simulink model "ue_tracking"  (R2020a)
settings: Solver=FixedStepDiscrete  StartTime=0.0  StopTime=300  FixedStep=system.step  RelTol=1e-3
undefined symbols (not defined in the file or in its folder): frame, physconst, system, UE
libraries: commsync2 x3, phasedtxrxlib x3, phaseddoalib x2, commsink2 x2, commdigbbndpm3 x2, commfilt2 x2, commsequence2 x2, phasedbflib x2, commchan3 x2, dspsrcs4 x1, commrfcorlib x1, commutil2 x1
settings Model: PauseTimes=500  NumberOfSteps=10  Creator=jose_  LastModifiedBy=jose_
settings DebuggingCC: ReadBeforeWriteMsg=DisableAll  WriteAfterWriteMsg=DisableAll  WriteAfterReadMsg=DisableAll  MultiTaskDSMMsg=none
settings ModelReferenceCC: UpdateModelReferenceTargets=IfOutOfDate
settings SFSimCC: SFSimEcho=off

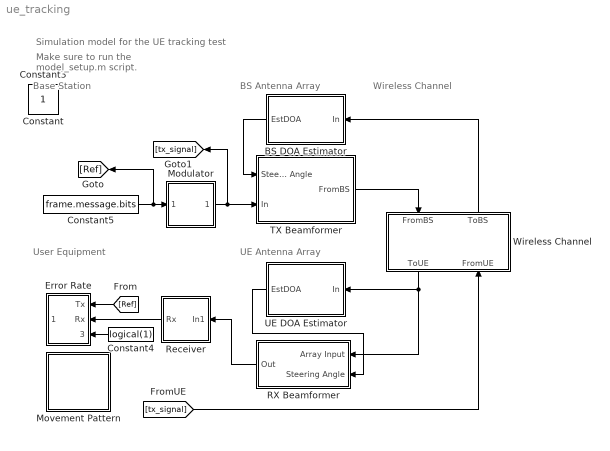
== system ue_tracking ==
  note: UE Antenna Array
  note: BS Antenna Array
  note: Wireless Channel
  note: User Equipment
  note: Base Station
  note: Make sure to run the model_setup.m script.
  note: Simulation model for the UE tracking test
  BS DOA Estimator : Subsystem
      mask Display: image('$imagefile'); % Use "Edit Image" on toolstrip to change.
  Constant4 : Constant  Value=logical(1)
  Constant5 : Constant  Value=frame.message.bits  SampleTime=system.step
  Error Rate : Subsystem
  Modulator : Subsystem
      mask Display: image('$imagefile'); % Use "Edit Image" on toolstrip to change.
  Movement Pattern : Subsystem
      mask Display: image('$imagefile'); % Use "Edit Image" on toolstrip to change.
  RX Beamformer : Subsystem
      mask Display: image('$imagefile'); % Use "Edit Image" on toolstrip to change.
  Receiver : Subsystem
      mask Display: image('$imagefile'); % Use "Edit Image" on toolstrip to change.
  TX Beamformer : Subsystem
      mask Display: image('$imagefile'); % Use "Edit Image" on toolstrip to change.
  UE DOA Estimator : Subsystem
      mask Display: image('$imagefile'); % Use "Edit Image" on toolstrip to change.
  Wireless Channel : Subsystem
      settings: PortSchema="{\"entries\":[{\"content\":{\"sides\":[{\"content\":{\"connectorIds\":[]},\"type\":\"ConnectorPlacement.EquallySpacedRectSide\",\"uuid\":\"75bf1423-5319-4e93-9a5f-3cb48862b48c\"},{\"content\":{\"connectorIds\":[],\"side\":\"RIGHT\"},\"type\":\"ConnectorPlacement.EquallySpacedRectSide\",\"uuid\":\"e5a97bb0-755e-4af0-92a4-b9cdae2be643\"},{\"content\":{\"connectorIds\":[\"In1\",\"Out2\"],\"side\":\"TOP\"},\"type\":\"ConnectorPlacement.EquallySpacedRectSide\",\"uuid\":\"177e5c48-1e85-4698-92ad-7f86d2203077\"},{\"content\":{\"connectorIds\":[\"Out1\",\"In2\"],\"side\":\"BOTTOM\"},\"type\":\"ConnectorPlacement.EquallySpacedRectSide\",\"uuid\":\"6d25e01a-df39-4651-afd4-30d22a581838\"}]},\"type\":\"ConnectorPlacement.EquallySpacedConnector\",\"uuid\":\"14e51280-45ab-4234-928d-dd2548344928\"}],\"packageUris\":[\"http://schema.mathworks.com/mf0/Connector/19700101\"],\"version\":\"1.0\"}"
      mask Display: image('$imagefile'); % Use "Edit Image" on toolstrip to change.
  Constant : Constant  IOType=siggen
  Constant3 : Constant  IOType=siggen
  wires:
  RX Beamformer/1(Out) -> Receiver/1(In1)
  Wireless Channel/2(ToBS) -> BS DOA Estimator/1(In)
  [tx_signal] -> Wireless Channel/2(FromUE)
  BS DOA Estimator/1(EstDOA) -> TX Beamformer/1(Steering Angle)
  Constant4/1 -> Error Rate/3(Rst)
  [Ref] -> Error Rate/1(Tx)
  Constant5/1 -> Modulator/1(Message), [Ref]
  Modulator/1(Out1) -> [tx_signal], TX Beamformer/2(In)
  Wireless Channel/1(ToUE) -> UE DOA Estimator/1(In), RX Beamformer/1(Array Input)
  Receiver/1(Rx) -> Error Rate/2(Rx)
  TX Beamformer/1(FromBS) -> Wireless Channel/1(FromBS)
  UE DOA Estimator/1(EstDOA) -> RX Beamformer/2(Steering Angle)

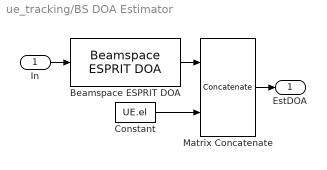
== system ue_tracking/BS DOA Estimator ==
  In : Inport
  Beamspace ESPRIT DOA : phaseddoalib/Beamspace ESPRIT DOA  PropagationSpeed=physconst( 'LightSpeed' )  OperatingFrequency=system.freq  NumSignalsSource=Property  NumSignalsMethod=AIC  NumSignals=1  SpatialSmoothing=0  Method=TLS  BeamFanCenter=0  NumBeamsSource=Auto  NumBeams=2  SimulateUsing=Code generation  SensorArray=AntennaArray
      settings: SourceProductBaseCode=AR
  Constant : Constant  Value=UE.el
  Matrix Concatenate : Concatenate  Mode=Multidimensional array
  EstDOA : Outport
  wires:
  In/1 -> Beamspace ESPRIT DOA/1
  Beamspace ESPRIT DOA/1 -> Matrix Concatenate/1
  Matrix Concatenate/1 -> EstDOA/1
  Constant/1 -> Matrix Concatenate/2

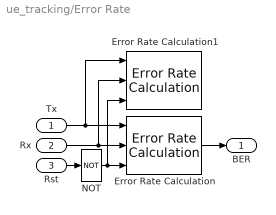
== system ue_tracking/Error Rate ==
  Tx : Inport
  Rx : Inport  Port=2
  Rst : Inport  Port=3
  Error Rate Calculation : commsink2/Error Rate Calculation  N=0  st_delay=0  cp_mode=Entire frame  subframe=[]  PMode=Port  WsName=ErrorVec  RsMode2=on  stop=off  numErr=100  maxBits=1e6
  Error Rate Calculation1 : commsink2/Error Rate Calculation  N=0  st_delay=0  cp_mode=Entire frame  subframe=[]  PMode=Workspace  WsName=ErrorVec  RsMode2=on  stop=off  numErr=100  maxBits=1e6
  NOT : Logic  Operator=NOT  IconShape=distinctive  AllPortsSameDT=off  OutDataTypeStr=boolean
  BER : Outport
  wires:
  Tx/1 -> Error Rate Calculation1/1, Error Rate Calculation/1
  Rx/1 -> Error Rate Calculation1/2, Error Rate Calculation/2
  Error Rate Calculation/1 -> BER/1
  Rst/1 -> NOT/1
  NOT/1 -> Error Rate Calculation1/3, Error Rate Calculation/3

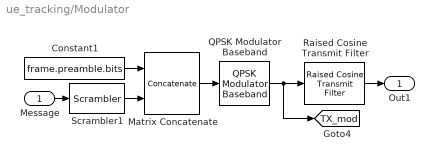
== system ue_tracking/Modulator ==
  Message : Inport
  Constant1 : Constant  Value=frame.preamble.bits  SampleTime=system.step
  Matrix Concatenate : Concatenate  Mode=Multidimensional array
  QPSK Modulator Baseband : commdigbbndpm3/QPSK Modulator Baseband  InType=Bit  Enc=Gray  Ph=system.mod.PhaseOffset  outDtype=double  outWordLen=16  outUDDataType=sfix(16)  outFracLenMode=Best precision  outFracLen=15  outDataTypeStr=double  outLastDataTypeStr=double
  Raised Cosine Transmit Filter : commfilt2/Raised Cosine Transmit Filter  filtType=Square root  R=system.tx.rc.rolloff  filtSpan=system.tx.rc.span  N=system.tx.rc.interpolation  filterGain=sqrt(system.tx.rc.interpolation)  InputProcessing=Columns as channels (frame based)  RateOptions=Enforce single-rate processing  framing=Mute  checkCoeff=off  variableName=rcTxFilt  checkGain=Normalized  sampMode=Mute  saveAsFlag=0  currentFiltSpan=system.tx.rc.span  D=(system.tx.rc.span)/2  launchFVT=on  roundingMode=Floor  overflowMode=off  coeffDataTypeStr=Inherit: Same word length as input  coeffMin=[]  coeffMax=[]  coeffLastDataTypeStr=Inherit: Same word length as input  outputDataTypeStr=Inherit: Same as accumulator  outputMin=[]  outputMax=[]  outputLastDataTypeStr=Inherit: Same as accumulator
  Scrambler1 : commsequence2/Scrambler  M=2  poly=[1 1 1 0 1]  iniStaSource=Dialog Parameter  ini_sta=[0 0 0 0]  resetViaPort=off
      settings: SourceProductBaseCode=CM
  Out1 : Outport
  tag scope: TX_mod=global
  wires:
  QPSK Modulator Baseband/1 -> [TX_mod], Raised Cosine Transmit Filter/1
  Matrix Concatenate/1 -> QPSK Modulator Baseband/1
  Raised Cosine Transmit Filter/1 -> Out1/1
  Constant1/1 -> Matrix Concatenate/1
  Message/1 -> Scrambler1/1
  Scrambler1/1 -> Matrix Concatenate/2

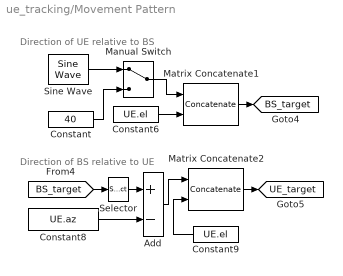
== system ue_tracking/Movement Pattern ==
  note: Direction of BS relative to UE
  note: Direction of UE relative to BS
  Add : Sum  Inputs=+-
  Constant : Constant  Value=40
  Constant6 : Constant  Value=UE.el  VectorParams1D=off
  Constant8 : Constant  Value=UE.az
  Constant9 : Constant  Value=UE.el  VectorParams1D=off
  Manual Switch : ManualSwitch
  Matrix Concatenate1 : Concatenate  Mode=Multidimensional array
  Matrix Concatenate2 : Concatenate  Mode=Multidimensional array
  Selector : Selector  InputPortWidth=2  IndexOptions=Index vector (dialog)  Indices=1  OutputSizes=1
  Sine Wave : dspsrcs4/Sine Wave  Amplitude=UE.max_ang  Frequency=UE.movement_freq  Phase=0  SampleMode=Discrete  OutComplex=Real  CompMethod=Table lookup  TableSize=Speed  SampleTime=system.step  SamplesPerFrame=1  ResetState=Restart at time zero  OutputFrames=off  dataType=double  wordLen=16  udDataType=sfix(16)  fracBitsMode=Best precision  numFracBits=15  OutDataTypeStr=double  LastOutDataTypeStr=double
  tag scope: BS_target=global, UE_target=global
  wires:
  Constant6/1 -> Matrix Concatenate1/2
  [BS_target] -> Selector/1
  Constant8/1 -> Add/2
  Matrix Concatenate2/1 -> [UE_target]
  Constant9/1 -> Matrix Concatenate2/2
  Matrix Concatenate1/1 -> [BS_target]
  Sine Wave/1 -> Manual Switch/1
  Constant/1 -> Manual Switch/2
  Manual Switch/1 -> Matrix Concatenate1/1
  Selector/1 -> Add/1
  Add/1 -> Matrix Concatenate2/1

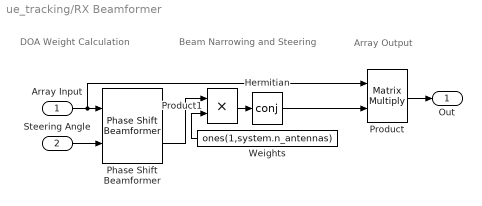
== system ue_tracking/RX Beamformer ==
  note: Beam Narrowing and Steering
  note: DOA Weight Calculation
  note: Array Output
  Array Input : Inport
  Steering Angle : Inport  Port=2
  Hermitian : Math  Operator=conj  SaturateOnIntegerOverflow=on
  Phase Shift Beamformer : phasedbflib/Phase Shift Beamformer  PropagationSpeed=physconst( 'LightSpeed' )  OperatingFrequency=system.freq  DirectionSource=Input port  Direction=[ 0; 0 ]  NumPhaseShifterBits=0  WeightsNormalization=Preserve power  WeightsOutputPort=on  SimulateUsing=Code generation  SensorArray=AntennaArray
      settings: SourceProductBaseCode=AR
  Product : Product  Multiplication=Matrix(*)
  Product1 : Product
  Weights : Constant  Value=ones(1,system.n_antennas)
  Out : Outport
  wires:
  Product1/1 -> Hermitian/1
  Hermitian/1 -> Product/2
  Product/1 -> Out/1
  Weights/1 -> Product1/2
  Phase Shift Beamformer/2 -> Product1/1
  Array Input/1 -> Product/1, Phase Shift Beamformer/1
  Steering Angle/1 -> Phase Shift Beamformer/2

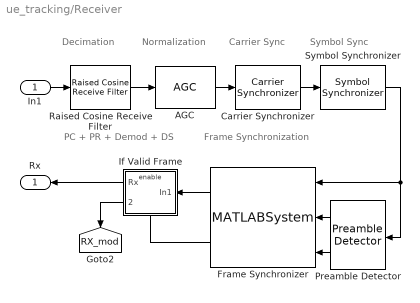
== system ue_tracking/Receiver ==
  note: PC + PR + Demod + DS
  note: Frame Synchronization
  note: Symbol Sync
  note: Carrier Sync
  note: Normalization
  note: Decimation
  In1 : Inport
  AGC : commrfcorlib/AGC  LegacyMode=off  DetectorMethod=Rectifier  LoopMethod=Linear  UpdatePeriod=100  StepSize=0.1  AdaptationStepSize=system.rx.agc.step  DesiredOutputPower=system.rx.agc.output_power  AveragingLength=system.rx.agc.average_length  MaximumGain=30  MaxPowerGain=system.rx.agc.max_power  GainOutputPort=off  InputPowerOutputPort=off  SimulateUsing=Code generation
  Carrier Synchronizer : commsync2/Carrier Synchronizer  Modulation=QPSK  ModulationPhaseOffset=Auto  CustomPhaseOffset=0  SamplesPerSymbol=system.rx.cs.sps  DampingFactor=system.rx.cs.damp  NormalizedLoopBandwidth=system.rx.cs.bandwidth  EstimatedPhaseErrorOutputPort=off  SimulateUsing=Code generation
  Frame Synchronizer : MATLABSystem  System=comm.internal.examples.FrameSynchronizer  Input=Symbol  OutputFrameLength=system.rx.fs.frame_length  PreambleLength=system.rx.fs.preamble_length  SimulateUsing=Code generation
      mask Type: comm.internal.examples.FrameSynchronizer
      mask Display:
      | disp(['Frame' char(10) 'Synchronizer']);
      | port_label('input',1,'u');
      | port_label('input',2,'idx');
      | port_label('input',3,'dtMt');
      | port_label('output',1,'Frame');
      | port_label('output',2,'Valid');
  If Valid Frame : Subsystem  TreatAsAtomicUnit=on
  Preamble Detector : commsync2/Preamble Detector  Input=Symbol  Preamble=system.rx.pd.preamble  Threshold=system.rx.pd.threshold  DetectionMetricOutput=on  Detections=All  SimulateUsing=Code generation
      settings: SourceProductBaseCode=CM
  Raised Cosine Receive Filter : commfilt2/Raised Cosine Receive Filter  filtType=Square root  R=system.rx.rc.rolloff  filtSpan=system.rx.rc.span  N=system.rx.rc.sps  downFactor=system.rx.rc.decimation  downOffset=0  filterGain=1/sqrt(10)  InputProcessing=Columns as channels (frame based)  RateOptions=Enforce single-rate processing  framing=Mute  checkCoeff=off  variableName=rcRxFilt  currentFiltSpan=system.rx.rc.span  D=(system.rx.rc.span)/2  inputOffset=0  sampMode=Mute  saveAsFlag=0  rateMode=Downsampling  checkGain=Normalized  launchFVT=on  roundingMode=Floor  overflowMode=off  coeffDataTypeStr=Inherit: Same word length as input  coeffMin=[]  coeffMax=[]  coeffLastDataTypeStr=Inherit: Same word length as input  accumDataTypeStr=Inherit: Same as product output  accumLastDataTypeStr=Inherit: Same as product output  outputDataTypeStr=Inherit: Same as accumulator  outputMin=[]  outputMax=[]  outputLastDataTypeStr=Inherit: Same as accumulator
  Symbol Synchronizer : commsync2/Symbol Synchronizer  Modulation=PAM/PSK/QAM  TimingErrorDetector=Zero-Crossing (decision-directed)  SamplesPerSymbol=system.rx.ss.sps  DampingFactor=system.rx.ss.damp  NormalizedLoopBandwidth=system.rx.ss.bandwidth  DetectorGain=system.rx.ss.gain  TimingErrorOutputPort=off  SimulateUsing=Code generation
      settings: SourceProductBaseCode=CM
  Rx : Outport
  tag scope: RX_mod=global
  wires:
  In1/1 -> Raised Cosine Receive Filter/1
  Raised Cosine Receive Filter/1 -> AGC/1
  Preamble Detector/1 -> Frame Synchronizer/2
  Frame Synchronizer/1 -> If Valid Frame/1(In1)
  If Valid Frame/1(Rx) -> Rx/1
  Frame Synchronizer/2 -> If Valid Frame/Enable
  AGC/1 -> Carrier Synchronizer/1
  Carrier Synchronizer/1 -> Symbol Synchronizer/1
  Preamble Detector/2 -> Frame Synchronizer/3
  Symbol Synchronizer/1 -> Frame Synchronizer/1, Preamble Detector/1
  If Valid Frame/2(pre-demod) -> [RX_mod]

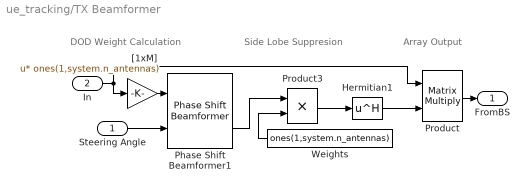
== system ue_tracking/TX Beamformer ==
  note: Array Output
  note: Side Lobe Suppresion
  note: DOD Weight Calculation
  Steering Angle : Inport
  In : Inport  Port=2
  Hermitian1 : Math  Operator=hermitian  SaturateOnIntegerOverflow=on
  Phase Shift Beamformer1 : phasedbflib/Phase Shift Beamformer  PropagationSpeed=physconst( 'LightSpeed' )  OperatingFrequency=system.freq  DirectionSource=Input port  Direction=[ 0; 0 ]  NumPhaseShifterBits=0  WeightsNormalization=Preserve power  WeightsOutputPort=on  SimulateUsing=Code generation  SensorArray=AntennaArray
      settings: SourceProductBaseCode=AR
  Product : Product  Multiplication=Matrix(*)
  Product3 : Product
  Weights : Constant  Value=ones(1,system.n_antennas)  SampleTime=system.step
  "[1xM]" : Gain  Gain=ones(1,system.n_antennas)  Multiplication=Matrix(u*K)
  FromBS : Outport
  wires:
  Weights/1 -> Product3/2
  Phase Shift Beamformer1/2 -> Product3/1
  Steering Angle/1 -> Phase Shift Beamformer1/2
  Hermitian1/1 -> Product/2
  Product3/1 -> Hermitian1/1
  Product/1 -> FromBS/1
  In/1 -> "[1xM]"/1, Product/1
  "[1xM]"/1 -> Phase Shift Beamformer1/1

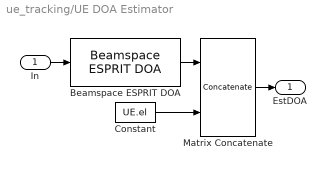
== system ue_tracking/UE DOA Estimator ==
  In : Inport
  Beamspace ESPRIT DOA : phaseddoalib/Beamspace ESPRIT DOA  PropagationSpeed=physconst( 'LightSpeed' )  OperatingFrequency=system.freq  NumSignalsSource=Property  NumSignalsMethod=AIC  NumSignals=1  SpatialSmoothing=0  Method=TLS  BeamFanCenter=0  NumBeamsSource=Auto  NumBeams=1  SimulateUsing=Code generation  SensorArray=AntennaArray
      settings: SourceProductBaseCode=AR
  Constant : Constant  Value=UE.el
  Matrix Concatenate : Concatenate  Mode=Multidimensional array
  EstDOA : Outport
  wires:
  In/1 -> Beamspace ESPRIT DOA/1
  Beamspace ESPRIT DOA/1 -> Matrix Concatenate/1
  Matrix Concatenate/1 -> EstDOA/1
  Constant/1 -> Matrix Concatenate/2

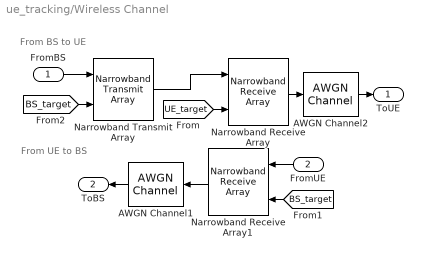
== system ue_tracking/Wireless Channel ==
  note: From UE to BS
  note: From BS to UE
  FromBS : Inport
  FromUE : Inport  Port=2
  AWGN Channel1 : commchan3/AWGN Channel  InputProcessing=Columns as channels (frame based)  seed=25  noiseMode="Signal to noise ratio  (Eb/No)"  EbNodB=channel.snr  EsNodB=10  SNRdB=EbNo  bitsPerSym=2  Ps=1  Tsym=system.step/length(frame.symbols)  variance=1
  AWGN Channel2 : commchan3/AWGN Channel  InputProcessing=Columns as channels (frame based)  seed=25  noiseMode="Signal to noise ratio  (Eb/No)"  EbNodB=channel.snr  EsNodB=10  SNRdB=EbNo  bitsPerSym=2  Ps=1  Tsym=system.step/length(frame.symbols)  variance=1
  Narrowband Receive Array : phasedtxrxlib/Narrowband Receive Array  PropagationSpeed=physconst( 'LightSpeed' )  OperatingFrequency=system.freq  Wavefront=Plane  SensorGainMeasure=dB  Polarization=None  WeightsInputPort=off  SimulateUsing=Code generation  Sensor=AntennaArray
      settings: SourceProductBaseCode=AR
  Narrowband Receive Array1 : phasedtxrxlib/Narrowband Receive Array  PropagationSpeed=physconst( 'LightSpeed' )  OperatingFrequency=system.freq  Wavefront=Plane  SensorGainMeasure=dB  Polarization=None  WeightsInputPort=off  SimulateUsing=Code generation  Sensor=AntennaArray
      settings: SourceProductBaseCode=AR
  Narrowband Transmit Array : phasedtxrxlib/Narrowband Transmit Array  PropagationSpeed=physconst( 'LightSpeed' )  OperatingFrequency=system.freq  CombineRadiatedSignals=on  SensorGainMeasure=dB  Polarization=None  WeightsInputPort=off  SimulateUsing=Code generation  Sensor=AntennaArray
      settings: SourceProductBaseCode=AR
  ToUE : Outport
  ToBS : Outport  Port=2
  wires:
  AWGN Channel2/1 -> ToUE/1
  [UE_target] -> Narrowband Receive Array/2
  Narrowband Receive Array1/1 -> AWGN Channel1/1
  FromUE/1 -> Narrowband Receive Array1/1
  AWGN Channel1/1 -> ToBS/1
  [BS_target] -> Narrowband Receive Array1/2
  [BS_target] -> Narrowband Transmit Array/2
  FromBS/1 -> Narrowband Transmit Array/1
  Narrowband Transmit Array/1 -> Narrowband Receive Array/1
  Narrowband Receive Array/1 -> AWGN Channel2/1

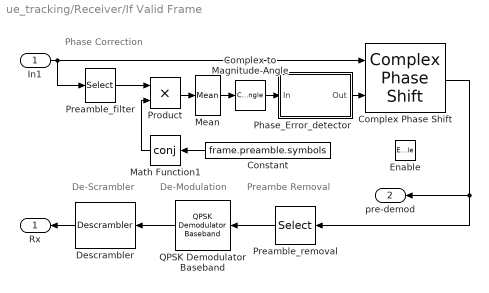
== system ue_tracking/Receiver/If Valid Frame ==
  note: De-Scrambler
  note: De-Modulation
  note: Preambe Removal
  note: Phase Correction
  In1 : Inport
  Enable : EnablePort
  Complex Phase Shift : commutil2/Complex Phase Shift
      settings: SourceProductBaseCode=CM
  Complex to Magnitude-Angle : ComplexToMagnitudeAngle  Output=Angle
  Constant : Constant  Value=frame.preamble.symbols
  Descrambler : commsequence2/Descrambler  M=2  poly=[1 1 1 0 1]  iniStaSource=Dialog Parameter  ini_sta=[0 0 0 0]  resetViaPort=off
      settings: SourceProductBaseCode=CM
  Math Function1 : Math  Operator=conj  SignedPower=on  SaturateOnIntegerOverflow=on
  Mean : dspstat3/Mean  run=off  InputProcessing=Columns as channels (frame based)  reset_popup=None  directionMode=Each column  dimension=1  roiEnable=off  roiType=Rectangles  roiPortion=Entire ROI  roiOutput=Individual statistics for each ROI  roiFlag=off  roundingMode=Floor  overflowMode=off  outputDataTypeStr=Inherit: Same as accumulator  outputMin=[]  outputMax=[]  outputLastDataTypeStr=Inherit: Same as accumulator
  Phase_Error_detector : MATLAB Function  TreatAsAtomicUnit=on
  Preamble_filter : Selector  InputPortWidth=length(frame.symbols)  IndexOptions=Index vector (dialog)  Indices=1:length(frame.preamble.symbols)  OutputSizes=1
  Preamble_removal : Selector  InputPortWidth=length(frame.symbols)  IndexOptions=Index vector (dialog)  Indices=(length(frame.preamble.symbols)+1):length(frame.symbols)  OutputSizes=1
  Product : Product  RndMeth=Zero
  QPSK Demodulator Baseband : commdigbbndpm3/QPSK Demodulator Baseband  OutType=Bit  DecType=Hard decision  VarSource=Dialog  Variance=1  Dec=Gray  Ph=system.mod.PhaseOffset  outDtype1=Inherit via internal rule  outDtype2=Inherit via internal rule  derotateFactorWordLen=16  derotateFactorDataTypeStr=Inherit: Same word length as input  derotateFactorLastDataTypeStr=Inherit: Same word length as input
  Rx : Outport
  pre-demod : Outport  Port=2
  wires:
  Mean/1 -> Complex to Magnitude-Angle/1
  Product/1 -> Mean/1
  Complex to Magnitude-Angle/1 -> Phase_Error_detector/1(In)
  Preamble_filter/1 -> Product/1
  In1/1 -> Preamble_filter/1, Complex Phase Shift/1
  Constant/1 -> Math Function1/1
  Phase_Error_detector/1(Out) -> Complex Phase Shift/2
  Complex Phase Shift/1 -> Preamble_removal/1, pre-demod/1
  Math Function1/1 -> Product/2
  Preamble_removal/1 -> QPSK Demodulator Baseband/1
  QPSK Demodulator Baseband/1 -> Descrambler/1
  Descrambler/1 -> Rx/1

== matlab function ue_tracking/Receiver/If Valid Frame/Phase_Error_detector ==
  data: In input; Out output
function Out = phasedecision(In)
% Map the estimated phase to one of -pi, -pi/2, 0, pi/2,  
%#codegen
Out = -round(In.*2./pi)./2.*pi;
% The above processing is equivalent to the following processing using
% if/else statements
%
% if In<pi/4 && In>-pi/4
%     Out = 0;
% elseif In>=pi/4 && In<pi*3/4
%     Out = pi/2;
% elseif In>=pi*3/4 || In<=-pi*3/4
%     Out = -pi;
% else
%     Out = -pi/2;
% end
